simulink library "DAEMOT_Lib"  (R2019b)
settings: Solver=ode45  StartTime=0.0  StopTime=10.0  FixedStep=0.1  RelTol=1e-3
undefined symbols (not defined in the file or in its folder): Controller, CP, Ctrl, Ctrl_Fcn, Elec1, f, F2, Fluid, lag1, Mission, Moody, PropellerProp, rev_comms_sink
libraries: $bdroot x200, instrumentlib x21, simulink x5, dspsigops x2
(part 12 of 13)

== matlab function DAEMOT_Lib/Thermal/Heat Exchanger/HX ==
  data: x input; x_dot output; P_in input size=2; Mdot_down input size=2; Mdot input; T_in input size=2; H output; mu input size=2; k input size=2; Cp input size=2; Rho input size=2; E_fluid input size=2; M_wall parameter; Cp_wall parameter; Pass1 parameter; Pass2 parameter; f1 parameter; f2 parameter; KL1 parameter; KL2 parameter; b1 parameter; b2 parameter; W1 parameter; W2 parameter; L1 parameter; L2 parameter; Nu_lam1 parameter; Nu_lam2 parameter; dH1 parameter; dH2 parameter; HTC_method1 parameter; HTC_method2 parameter; HTC1 parameter; HTC2 parameter
function [x_dot,H]  = HX(x,P_in,Mdot_down,Mdot,T_in,mu,k,Cp,Rho,E_fluid,M_wall,Cp_wall,Pass1,Pass2,f1,f2,KL1,KL2,b1,b2,W1,W2,L1,L2,Nu_lam1,Nu_lam2,dH1,dH2,HTC_method1, HTC_method2, HTC1, HTC2)

% Parse data
P_in1       = P_in(1);
P_in2       = P_in(2);
Mdot_down1  = Mdot_down(1);
Mdot_down2  = Mdot_down(2);
Mdot1       = Mdot(1);
Mdot2       = Mdot(2);
T_in1       = T_in(1);
T_in2       = T_in(2);
mu1         = mu(1);
mu2         = mu(2);
k1          = k(1);
k2          = k(2);
Cp1         = Cp(1);
Cp2         = Cp(2);
Rho1        = Rho(1);
Rho2        = Rho(2);
E_fluid1    = E_fluid(1);
E_fluid2    = E_fluid(2);

% Constants and Conversions
Mdot_down1_pass = Mdot_down1/Pass1;
Mdot_down2_pass = Mdot_down2/Pass2;
Mdot1_pass = Mdot1/Pass1;
Mdot2_pass = Mdot2/Pass2;
g        = 9.81;                   % Gravitational acceleration [m/s^2]
A_ht1    = L1*(2*b1+2*W1);         % Heat transfer area
A_ht2    = L2*(2*b2+2*W2);         % Heat transfer area
V1       = L1*b1*W1;               % Volume per pass
V2       = L2*b2*W2;               % Volume per pass
Cp1      = 1000*Cp1;               % Convert Cp from J/g*K to J/kg*K
Cp2      = 1000*Cp2;               % Convert Cp from J/g*K to J/kg*K
k1       = 1000*k1;                % Convert k from kW/m*K to W/m*K
k2       = 1000*k2;                % Convert k from kW/m*K to W/m*K
C_wall   = M_wall*Cp_wall;         % Heat Capacitance (kJ/K)
C_wall   = 1000*C_wall;            % Covnert heat capacitance from kJ/K to J/K
D1       = 4*b1*W1/(2*b1+2*W1);    % Hydraulic diameter (side 1) (see Incropera, Eq. 8.66)
D2       = 4*b2*W2/(2*b2+2*W2);    % Hydraulic diameter (side 2) (see Incropera, Eq. 8.66)

% Parse states
Tw      = x(1);                 % Wall temperature
P1      = x(2);                 % Outlet pressure (side 1)
P2      = x(3);                 % Outlet pressure (side 2)
T1      = x(4);                 % Outlet temperature (side 1)
T2      = x(5);                 % Outlet temperature (side 2)

% Additional intermediate variable calculations
dP1         = (P_in1-P1)*1000;      % Pressure differential (side 1) [Pa]
dP2         = (P_in2-P2)*1000;      % Pressure differential (side 2) [Pa]
dP1         = dP1 + Rho1*g*dH1;     % Pressure differential corrected for hieght
dP2         = dP2 + Rho2*g*dH2;     % Pressure differential corrected for hieght
um1         = sign(dP1)*sqrt_Lip(2*abs(dP1)/(Rho1*(f1*L1/D1+KL1)));   % Fluid velocity (side 1) [m/s]
um2         = sign(dP2)*sqrt_Lip(2*abs(dP2)/(Rho2*(f2*L2/D2+KL2)));   % Fluid velocity (side 2) [m/s]
Re1         = Rho1*abs(um1)*D1/mu1;      % Reynolds number (side 1)
Re2         = Rho2*abs(um2)*D2/mu2;      % Reynolds number (side 1)
Pr1         = Cp1*mu1/k1;           % Prandtl number (side 1) (see Incropera, Table 6.2)
Pr2         = Cp2*mu2/k2;           % Prandtl number (side 2) (see Incropera, Table 6.2)

% Gneilinski
if Re1 < 2300
    Nu1 = Nu_lam1; % (inteprolated from Incropera, Table 8.1 in initialization)
else
    Nu1 = (f1/8)*(Re1-1000)*Pr1 / (1+12.7*(f1/8)^.5*(Pr1^(2/3)-1)); % (see Incropera, Eq. 8.62)
end
if Re2 < 2300
    Nu2 = Nu_lam2; % (inteprolated from Incropera, Table 8.1 in initialization)
else
    Nu2 = (f2/8)*(Re2-1000)*Pr2 / (1+12.7*(f2/8)^.5*(Pr2^(2/3)-1)); % (see Incropera, Eq. 8.62)
end

% Longo Correlation
% Nu1 = 0.277*Re1^0.766*Pr1^0.333;
% Nu2 = 0.277*Re2^0.766*Pr2^0.333;

% % Manglik Correlation
% Nu1 = 0.44*Re1^0.5*Pr1^0.333;
% Nu2 = 0.44*Re2^0.5*Pr2^0.333;

% Calculate outputs
if HTC_method1 == 0
    H1      = Nu1*k1/D1;        % Heat transfer coefficient (see Incropera, Table 6.2)
else
    H1 = HTC1;
end
if HTC_method2 == 0
    H2      = Nu2*k2/D2;        % Heat transfer coefficient (see Incropera, Table 6.2)
else
    H2 = HTC2;
end
H       = [H1 H2];

% Calculate state derivatives
Tw_dot = ( H1*A_ht1*(T1-Tw) + H2*A_ht2*(T2-Tw) )/C_wall;    % Wall temperature
P1_dot = (Mdot1_pass-Mdot_down1_pass)/(V1*Rho1/E_fluid1);   % Outlet pressure (side 1)
P2_dot = (Mdot2_pass-Mdot_down2_pass)/(V2*Rho2/E_fluid2);   % Outlet pressure (side 2)
Tout1_dot = (Mdot1_pass*(T_in1-T1)+H1*A_ht1/Cp1*(Tw-T1))/(V1*Rho1);   % Outlet temperature (side 1)
Tout2_dot = (Mdot2_pass*(T_in2-T2)+H2*A_ht2/Cp2*(Tw-T2))/(V2*Rho2);   % Outlet temperature (side 2)

% Mux state derivatives
x_dot  = [Tw_dot,P1_dot,P2_dot,Tout1_dot,Tout2_dot];

end

== matlab function DAEMOT_Lib/Legacy Components/Fluid Tank/Tank ==
  data: x input; x_dot output; Mdot_in input; Mdot_out input; T_in input; T_amb input; Cp input; M output; h output; Rho input; H parameter; D parameter; Pamb parameter
function [x_dot,M,h]= Tank(x,Mdot_in,Mdot_out,T_in,T_amb,Cp,Rho,H,D,Pamb)

% Constants and Conversions
A_cross = pi*D^2/4;             % Cross-sectional area
Cp      = 1000*Cp;              % Convert Cp from J/g*K to J/kg*K
g       = 9.81;                 % Gravitational acceleration

% Parse states
T      = x(1);                  % Temperature of the tank
P      = x(2);                  % Pressure at bottom of the tank

% Calculate outputs
h = 1000*(P-Pamb)/(Rho*g);      % Tank height
M = Rho*A_cross*h;              % Tank mass

% Additional intermediate variable calculations
A_ht    = pi*h*D;               % Heat transfer area          

% Calculate state derivatives
T_dot = (Mdot_in*(T_in-T)-H*A_ht*(T-T_amb)/Cp)/M;    % Tank temperature
P_dot  = (Mdot_in-Mdot_out)*g/(1000*A_cross);        % Tank pressure

% Mux state derivatives
x_dot  = [T_dot,P_dot];

end

== matlab function DAEMOT_Lib/Thermal/Pump/Pump ==
  data: x input; x_dot output; Mdot output; P_in input; T_in input; Power output; Mdot_down input; PWM input; E_fluid input; Rho input; D parameter; L parameter; t parameter; E parameter; v parameter; A input; H_k input; Rho_pump input; Eta_k input
function [x_dot,Mdot,Power]= Pump(x,P_in,T_in,Mdot_down,PWM,E_fluid,Rho,D,L,t,E,v,A,H_k,Rho_pump,Eta_k)


% Constants and Conversions
V           = L*pi*D^2/4;       % Volume
g           = 9.81;             % Gravitational acceleration

% Parse states
T       = x(1);                 % Temperature of the tank
P       = x(2);                 % Pressure at bottom of the tank

% Additional intermediate variable calculations
dP      = (P-P_in);             % Pressure difference [kPa]
PWM     = PWM/100;              % PWM in duty ratio [0-1]
H       = H_k' * [1; dP; PWM];   % Pump head [m]
Q       = sqrt_Lip( max(0,2*g*(H - 1000*dP/(Rho_pump*g))) )*A;  % Volumetric flow rate
WHP     = Rho*g*Q*H;            % Pump water horse power [W]
Eta     = Eta_k' * [1; WHP; PWM; WHP^2; PWM^2; WHP*PWM];   % Efficiency [%]

% Calculate outputs
Mdot    = Rho*Q;                % Mass flow rate [kg/s]
Power   = (Eta/100)*WHP;        % Pump electrical power [W]
         
% Calculate state derivatives
T_dot   = Mdot*(T_in-T)/(V*Rho);    % Pump outlet temperature 
P_dot   = (Mdot-Mdot_down)/(V*Rho*(1/E_fluid+D*(1-v/2)/(t*E))); % Pump outlet pressure

% Mux state derivatives
x_dot  = [T_dot,P_dot];

end

== matlab function DAEMOT_Lib/Legacy Components/Pipe_M_to_M/Pipe_M_to_M ==
  data: x input; x_dot output; Mdot_in input; Mdot_out input; Rho input; dRho_dP input; f input; D parameter; L parameter; P_in output; P_out output
function [x_dot,P_in,P_out] = Pipe_M_to_M(x,Mdot_in,Mdot_out,Rho,dRho_dP,f,D,L)

% Notes on Friction Factor:
% f is currently calculated using a lookup table generated with the "Hydro
% Scheme Designer" as: f  = moody(e/D,Re).  This Moody function
% automatically detects laminar vs. turbulent flow, but with a cutoff of 
% Re=2000.  This could lead to numerical issues in the future, as there is 
% a discrete transition in the lookup table at Re=2000 that could lead to
% oscillations about that point.

% Alternately, the code below could be used:
% f = (0.790*log(Re)-1.64)^-2; % (see Incropera, Eq. 8.21)
% if (Re<3000) || (Re>5*10^6)
%     disp('Reynolds Number is outside the range of the friction factor correlation.')
% end

mdot    = (Mdot_in+Mdot_out)/2; % Average mass flow rate
A_cross = pi*D^2/4;             % Cross-sectional area
V       = L*pi*D^2/4;           % Volume

% Parse states
P       = x(1);

% Calculate upstream and downstream pressure
L_diff  = L/2;
um      = mdot/(Rho*A_cross);
delta_P = (f*Rho*um^2/(2*D))*L_diff; % (see Incropera, Eq. 8.22a)
delta_P = delta_P/1000; % Convert from Pa to kPa
P_in    = P+delta_P;
P_out   = P-delta_P;

% Calculate state derivatives
P_dot   = (Mdot_in-Mdot_out)/(V*dRho_dP);

% Mux state derivatives
x_dot   = P_dot;

== matlab function DAEMOT_Lib/Thermal/Pipe_P_to_P/Pipe_P_to_M ==
  data: x_dot output; x input; T_in input; Mdot input; Rho input; D parameter; L parameter
function x_dot   = Pipe_P_to_M(x,T_in,Mdot,Rho,D,L)

% Constants and Conversions
V      = pi*D^2/4*L;            % Volume

% Parse states
T      = x(1);                  % Temperature of the tank

% Calculate state derivatives
T_dot  = Mdot*(T_in-T)/(V*Rho);  % Pipe outlet temperature

% Mux state derivatives
x_dot  = T_dot;

end

== matlab function DAEMOT_Lib/Thermal/Pipe_P_to_M/Pipe_P_to_M ==
  data: x_dot output; x input; T_in input; Mdot_down input; Mdot input; Rho input; E_fluid input; D parameter; L parameter; t parameter; E parameter; v parameter
function x_dot  = Pipe_P_to_M(x,T_in,Mdot_down,Mdot,Rho,E_fluid,D,L,t,E,v)

% Constants and Conversions
V       = L*pi*D^2/4;           % Volume

% Parse states
T       = x(1);                 % Temperature at the outlet of pipe
P       = x(2);                 % Pressure at the outlet of pipe

% Calculate state derivatives
T_dot = Mdot*(T_in-T)/(V*Rho);  % Pipe outlet temperature
P_dot = (Mdot-Mdot_down)/(V*Rho*(1/E_fluid+D*(1-v/2)/(t*E)));   % Pipe outlet pressure

% Mux state derivatives
x_dot  = [T_dot,P_dot];

end

== matlab function DAEMOT_Lib/Thermal/Pipe_P_to_M/Mdot ==
  data: P_in input; P_out input; Mdot output; Rho input; f parameter; D parameter; L parameter; KL parameter; dH parameter
function Mdot = Mdot(P_in,P_out,Rho,f,D,L,KL,dH)

% Constants and Conversions
g           = 9.81;                 % Gravitational acceleration [m/s^2]
A_cross     = pi*D^2/4;             % Cross sectional area
dP          = (P_in-P_out)*1000;    % Pressure differential [Pa]
dP          = dP + Rho*g*dH;        % Pressure differential corrected for hieght
um          = max(0,sign(dP)*sqrt_Lip(2*abs(dP)/(Rho*(f*L/D+KL))));    % Fluid velocity [m/s]

% Calculate outputs
Mdot        = um*Rho*A_cross;       % Mass flow rate [kg/s]

end

== matlab function DAEMOT_Lib/Legacy Components/Pipe_M_to_P/Pipe_P_to_M ==
  data: x_dot output; x input; P_out input; Mdot_up input; Mdot output; Rho input; dRho_dP input; f input; D parameter; L parameter
function [x_dot,Mdot]  = Pipe_P_to_M(x,P_out,Mdot_up,Rho,dRho_dP,f,D,L)

% Notes on Friction Factor:
% f is currently calculated using a lookup table generated with the "Hydro
% Scheme Designer" as: f  = moody(e/D,Re).  This Moody function
% automatically detects laminar vs. turbulent flow, but with a cutoff of 
% Re=2000.  This could lead to numerical issues in the future, as there is 
% a discrete transition in the lookup table at Re=2000 that could lead to
% oscillations about that point.

% Alternately, the code below could be used:
% f = (0.790*log(Re)-1.64)^-2; % (see Incropera, Eq. 8.21)
% if (Re<3000) || (Re>5*10^6)
%     disp('Reynolds Number is outside the range of the friction factor correlation.')
% end

% Perform various conversions
A_cross = pi*D^2/4;                % Cross-sectional area
V       = L*pi*D^2/4;              % Volume

% Parse states
P_in  = x;

% Calculate mass flow rate
dP       = (P_in-P_out)*1000;
um       = sign(dP)*sqrt(4*abs(dP)*D/(L*Rho*f));
Mdot     = um*Rho*A_cross;

% Calculate state derivatives
P_dot  = (Mdot_up-Mdot)/(V*dRho_dP);

% Mux state derivatives
x_dot  = P_dot;

== matlab function DAEMOT_Lib/Thermal/Pipe_P_to_P/Mdot ==
  data: P_in input; P_out input; Mdot output; Rho input; f parameter; D parameter; L parameter; KL parameter; dH parameter
function Mdot = Mdot(P_in,P_out,Rho,f,D,L,KL,dH)

% Constants and Conversions
g           = 9.81;                 % Gravitational acceleration [m/s^2]
A_cross     = pi*D^2/4;             % Cross sectional area
dP          = (P_in-P_out)*1000;    % Pressure differential [Pa]
dP          = dP + Rho*g*dH;        % Pressure differential corrected for hieght
um          = max(0,sign(dP)*sqrt_Lip(2*abs(dP)/(Rho*(f*L/D+KL))));    % Fluid velocity [m/s]

% Calculate outputs
Mdot        = um*Rho*A_cross;       % Mass flow rate [kg/s]

end

== matlab function DAEMOT_Lib/Thermal/Heat Exchanger/Mdot ==
  data: P_in1 input; P_in2 input; Mdot1_tot output; P_out1 input; P_out2 input; Rho1 input; Rho2 input; f1 parameter; f2 parameter; b1 parameter; b2 parameter; W1 parameter; W2 parameter; L1 parameter; L2 parameter; KL1 parameter; KL2 parameter; Mdot2_tot output; Pass1 parameter; Pass2 parameter; dH1 parameter; dH2 parameter
function [Mdot1_tot,Mdot2_tot]   = Mdot(P_in1,P_in2,P_out1,P_out2,Rho1,Rho2,f1,f2,b1,b2,W1,W2,L1,L2,KL1,KL2,Pass1,Pass2,dH1,dH2)

% Constants and Conversions
g           = 9.81;                 % Gravitational acceleration [m/s^2]
D1 = 4*b1*W1/(2*b1+2*W1);           % (see Incropera, Eq. 8.66)
D2 = 4*b2*W2/(2*b2+2*W2);           % (see Incropera, Eq. 8.66)
dP1         = (P_in1-P_out1)*1000;  % Pressure differential (side 1) [Pa]
dP2         = (P_in2-P_out2)*1000;  % Pressure differential (side 2) [Pa]
dP1         = dP1 + Rho1*g*dH1;     % Pressure differential corrected for hieght
dP2         = dP2 + Rho2*g*dH2;     % Pressure differential corrected for hieght
um1         = max(0,sign(dP1)*sqrt_Lip(2*abs(dP1)/(Rho1*(f1*L1/D1+KL1)))); % Fluid velocity (side 1) [m/s]
um2         = max(0,sign(dP2)*sqrt_Lip(2*abs(dP2)/(Rho2*(f2*L2/D2+KL2)))); % Fluid velocity (side 2) [m/s]
Mdot1_pass  = um1*Rho1*b1*W1;       % Mass flow rate per pass (side 1) [kg/s]
Mdot2_pass  = um2*Rho2*b2*W2;       % Mass flow rate per pass (side 2) [kg/s]

% Calculate outputs
Mdot1_tot = Mdot1_pass*Pass1;       % Total mass flow rate (side 1) [kg/s]
Mdot2_tot = Mdot2_pass*Pass2;       % Total mass flow rate (side 2) [kg/s]

end

== matlab function DAEMOT_Lib/Legacy Components/Pipe_P_to_M1/Mdot ==
  data: P_in input; P_out input; Mdot output; Rho input; f parameter; D parameter; L parameter; KL parameter; dH parameter
function Mdot = Mdot(P_in,P_out,Rho,f,D,L,KL,dH)

% Constants and Conversions
g           = 9.81;                 % Gravitational acceleration [m/s^2]
A_cross     = pi*D^2/4;             % Cross sectional area
dP          = (P_in-P_out)*1000;    % Pressure differential [Pa]
dP          = dP + Rho*g*dH;        % Pressure differential corrected for hieght
um          = sign(dP)*sqrt(2*abs(dP)/(Rho*(f*L/D+KL)));    % Fluid velocity [m/s]

% Calculate outputs
Mdot        = um*Rho*A_cross;       % Mass flow rate [kg/s]

end

== matlab function DAEMOT_Lib/Legacy Components/Pipe_P_to_M1/Pipe_P_to_M ==
  data: x_dot output; x input; T_in input; Mdot_down input; Mdot input; Rho input; E_fluid input; D parameter; L parameter; t parameter; E parameter; v parameter
function x_dot  = Pipe_P_to_M(x,T_in,Mdot_down,Mdot,Rho,E_fluid,D,L,t,E,v)

% Constants and Conversions
V      = pi*D^2/4*L;            % Volume

% Parse states
T       = x(1);                 % Temperature at the outlet of pipe
P       = x(2);                 % Pressure at the outlet of pipe

% Calculate state derivatives
T_dot = Mdot*(T_in-T)/(V*Rho);  % Pipe outlet temperature
P_dot = (Mdot-Mdot_down)/(V*Rho*(1/E_fluid+D*(1-v/2)/(t*E)));   % Pipe outlet pressure

% Mux state derivatives
x_dot  = [T_dot,P_dot];

end

== matlab function DAEMOT_Lib/Legacy Components/Pipe_P_to_P1/Mdot ==
  data: P_in input; P_out input; Mdot output; Rho input; f parameter; D parameter; L parameter; KL parameter; dH parameter
function Mdot = Mdot(P_in,P_out,Rho,f,D,L,KL,dH)

% Constants and Conversions
g           = 9.81;                 % Gravitational acceleration [m/s^2]
A_cross     = pi*D^2/4;             % Cross sectional area
dP          = (P_in-P_out)*1000;    % Pressure differential [Pa]
dP          = dP + Rho*g*dH;        % Pressure differential corrected for hieght
um          = sign(dP)*sqrt(2*abs(dP)/(Rho*(f*L/D+KL)));    % Fluid velocity [m/s]

% Calculate outputs
Mdot        = um*Rho*A_cross;       % Mass flow rate [kg/s]

end

== matlab function DAEMOT_Lib/Legacy Components/Pipe_P_to_P1/Pipe_P_to_M ==
  data: x_dot output; x input; T_in input; Mdot input; Rho input; D parameter; L parameter
function x_dot   = Pipe_P_to_M(x,T_in,Mdot,Rho,D,L)

% Constants and Conversions
V      = pi*D^2/4*L;            % Volume

% Parse states
T      = x(1);                  % Temperature of the tank

% Calculate state derivatives
T_dot  = Mdot*(T_in-T)/(V*Rho);  % Pipe outlet temperature

% Mux state derivatives
x_dot  = T_dot;

end

== matlab function DAEMOT_Lib/Legacy Components/Solenoid_P_to_P/Mdot ==
  data: P_in input; P_out input; Mdot output; Rho input; f parameter; D parameter; L parameter; KL parameter
function Mdot = Mdot(P_in, P_out, Rho, f, D, L, KL)

% Constants and Conversions
A_cross     = pi*D^2/4;             % Cross sectional area
dP          = (P_in-P_out)*1000;    % Pressure differential [Pa]
um          = max(1e-6,sign(dP)*sqrt_Lip(2*abs(dP)/(Rho*(f*L/D+KL))));    % Fluid velocity [m/s]

% Calculate outputs
Mdot        = um*Rho*A_cross;       % Mass flow rate [kg/s]

end

== matlab function DAEMOT_Lib/Legacy Components/Solenoid_P_to_P/Pipe_P_to_M ==
  data: x_dot output; x input; T_in input; Mdot input; Rho input; D parameter; L parameter
function x_dot   = Solenoid_P_to_P(x,T_in,Mdot,Rho,D,L)

% Constants and Conversions
V      = pi*D^2/4*L;            % Volume

% Parse states
T      = x(1);                  % Temperature of the tank

% Calculate state derivatives
T_dot  = Mdot*(T_in-T)/(V*Rho);  % Pipe outlet temperature

% Mux state derivatives
x_dot  = T_dot;

end

== matlab function DAEMOT_Lib/Legacy Components/Solenoid_P_to_M/Mdot ==
  data: P_in input; P_out input; Mdot output; Rho input; f parameter; D parameter; L parameter; KL parameter
function Mdot = Mdot(P_in,P_out,Rho,f,D,L,KL)

% Constants and Conversions
A_cross     = pi*D^2/4;             % Cross sectional area
dP          = (P_in-P_out)*1000;    % Pressure differential [Pa]
um          = max(1e-6,sign(dP)*sqrt_Lip(2*abs(dP)/(Rho*(f*L/D+KL))));    % Fluid velocity [m/s]

% Calculate outputs
Mdot        = um*Rho*A_cross;       % Mass flow rate [kg/s]

end

== matlab function DAEMOT_Lib/Legacy Components/Solenoid_P_to_M/Pipe_P_to_M ==
  data: x_dot output; x input; T_in input; Mdot_down input; Mdot input; Rho input; E_fluid input; D parameter; L parameter; t parameter; E parameter; v parameter
function x_dot  = Solenoid_P_to_M(x,T_in,Mdot_down,Mdot,Rho,E_fluid,D,L,t,E,v)

% Constants and Conversions
V       = L*pi*D^2/4;           % Volume

% Parse states
T       = x(1);                 % Temperature at the outlet of pipe
P       = x(2);                 % Pressure at the outlet of pipe

% Calculate state derivatives
T_dot = Mdot*(T_in-T)/(V*Rho);  % Pipe outlet temperature
P_dot = (Mdot-Mdot_down)/(V*Rho*(1/E_fluid+D*(1-v/2)/(t*E)));   % Pipe outlet pressure

% Mux state derivatives
x_dot  = [T_dot,P_dot];

end

== matlab function DAEMOT_Lib/Thermal/Multi-Port Fluid Tank/Tank ==
  data: x input; x_dot output; Mdot_in input; Mdot_out input; T_in input; T_amb input; Cp input; M output; h output; Rho input; H parameter; D parameter; Pamb parameter
function [x_dot,M,h]= Tank(x,Mdot_in,Mdot_out,T_in,T_amb,Cp,Rho,H,D,Pamb)

% Constants and Conversions
Mdot_in_tot     = sum(Mdot_in);     % Total mass flow rate in
Mdot_out_tot    = sum(Mdot_out);    % Total mass flow rate out
A_cross = pi*D^2/4;             % Cross-sectional area
Cp      = 1000*Cp;              % Convert Cp from J/g*K to J/kg*K
g       = 9.81;                 % Gravitational acceleration

% Parse states
T      = x(1);                  % Temperature of the tank
P      = x(2);                  % Pressure at bottom of the tank

% Calculate outputs
h = 1000*(P-Pamb)/(Rho*g);      % Tank height
M = Rho*A_cross*h;              % Tank mass

% Additional intermediate variable calculations
A_ht    = pi*h*D;               % Heat transfer area          

% Calculate state derivatives
T_dot = ((dot(Mdot_in,T_in)-sum(Mdot_in)*T)-H*A_ht*(T-T_amb)/Cp)/M;    % Tank temperature
P_dot  = (Mdot_in_tot-Mdot_out_tot)*g/(1000*A_cross);        % Tank pressure

% Mux state derivatives
x_dot  = [T_dot,P_dot];

end

== matlab function DAEMOT_Lib/Legacy Components/Generator/Generator ==
  data: Omega input; I input; Torque output; V parameter; eta parameter; Q output
function [Torque,Q]   = Generator(Omega,I,V,eta)

% Constants and Conversions

% Parse states

% Additional intermediate variable calculations

% Calculate outputs
Torque = 1/(Omega*eta)*I*V;     % Generator torque (Nm)
Q = (1-eta)*Torque*Omega/1000;       % Generator heat (kW)

% Calculate state derivatives

% Mux state derivatives

end

== matlab function DAEMOT_Lib/Legacy Components/Aircraft/Aircraft ==
  data: x input; x_dot output; Thrust_1 input; Thrust_2 input; M_fuel input; M_dry parameter; M_load parameter; rho parameter; A parameter; Cd parameter
function x_dot = Aircraft(x,Thrust_1,Thrust_2,M_fuel,M_dry, M_load, rho, A, Cd)

% Parse states
Vel      = x(1);                  % Velocity of aircraft

% Additional intermediate variable calculations
M_tot  = M_fuel+M_dry+M_load;   % Total mass
Drag   = 0.5*rho*A*Cd*Vel^2;      % Drag force

% Calculate state derivatives
V_dot  = 1/(M_tot)*(Thrust_1+Thrust_2-Drag);    % Velocity

% Mux state derivatives
x_dot  = [V_dot];

end

== matlab function DAEMOT_Lib/Legacy Components/Engine/Engine ==
  data: x input; Mdot input; Vel input; Torque input; U input; x_dot output; Thrust output; J parameter; Thrust_max parameter; Omega_max parameter; Q_bearings output; alpha parameter; eta parameter
function [x_dot,Thrust,Q_bearings]  = Engine(x,Mdot,Vel,Torque,U,J,Thrust_max,Omega_max, alpha, eta)

% Constants and Conversions

% Parse states
Omega     = x(1);                 % Shaft Speed

% Additional intermediate variable calculations

% Calculate outputs
Thrust    = Thrust_max*(Omega/Omega_max)^3;  % Engine Thrust [N]
Q_burn    = (1-eta)*U*Mdot;           % Heat generation (leaves engine with exhaust) [kW]
Q_bearings = alpha*Omega;               % Bearing heat generation (cooled by oil) [kW]

% Calculate state derivatives
Omega_dot = 1/(J*Omega)*(1000*U*Mdot-Thrust*Vel-Torque*Omega-1000*(Q_burn+Q_bearings));    % Shaft speed 

% Mux state derivatives
x_dot  = [Omega_dot];

end

== matlab function DAEMOT_Lib/Thermal/Peristaltic_Pump/MATLAB Function ==
  data: P input; mdot output; w input; H_k input
% Calibration equations for drain pump 1 and drain pump 2 operating
% together at the same pump speed
% See 'Peristaltic Pump Flow Rates New Config.xlsx'

% mdot, kg/s - combined mass flow rate through both drain pumps
% w, [0-10] - drain pump speed (both drain pumps operate at same speed
% P, kPa - pressure at drain pumps

% Map for mdot was created Support Functions folder and raw data is
% in sensor calibration folder

function mdot = DrainPump(P, w, H_k)

mdot = any(w)*H_k(1) + H_k(2)*w + any(w)*H_k(3)*P;

% mdot = -0.0003743277602398326 + 0.00015072862953603*w + ...
%     0.00000307012873321525*P;
    
end

== matlab function DAEMOT_Lib/Legacy Components/Battery/Battery ==
  data: x input; V_in input; P input; x_dot output; I_in output; Q output; eta input; C parameter
function [x_dot,I_in,Q]  = Battery(x,V_in,P,eta,C)

% Constants and Conversions

% Parse states
SOC     = x(1);                 % State of charge

% Additional intermediate variable calculations

% Calculate outputs
if P >= 0   % Charge mode
    P_in = 1/eta*P;
    Q = (1-eta)*P_in;
else        % Discharge mode
    P_in = eta*P;
    Q = -(1-eta)*P;
end
I_in = 1000*P_in/V_in;

% Calculate state derivatives
SOC_dot = 1/(1000*C)*P;    % State of charge

% Mux state derivatives
x_dot  = [SOC_dot];

end

== matlab function DAEMOT_Lib/Electrical/Battery/Electrical ==
  data: I input; V input; T_m input; V1_dot output; props input size=[1 7]; B_cap parameter; V2_dot output; SOC_dot output; V_T output; Q output; Np parameter; Ns parameter
function [V1_dot,V2_dot,SOC_dot,V_T,Q]= Electrical(I,V,T_m,props,B_cap, Np,Ns)
%% Electrical Effects Function
Rs = props(1)*Ns/Np;
R1 = props(2)*Ns/Np;
C1 = props(3)*Np/Ns;
R2 = props(4)*Ns/Np;
C2 = props(5)*Np/Ns;
dU_dt = props(6)*Ns;
V_ocv = props(7);
V1 = V(1);
V2 = V(2);
%outputs = zeros(1,5);

%% Voltage Dynamics
V1_dot = -V1/(R1*C1) + I/C1;
V2_dot = -V2/(R2*C2) + I/C2;

%% State of Charge Dynamic
SOC_dot = -I/(3600*B_cap*Np);

%% Terminal Voltage
V_T = V_ocv - V1 - V2 - I*Rs;

%% Heat Generation
Q_s = (T_m+273)*dU_dt/1000; %entropic heat
Q = I^2*Rs + V1^2/R1 + V2^2/R2 - I*Q_s/Np;

== matlab function DAEMOT_Lib/Legacy Components/Converter/Converter ==
  data: V_in input; I input; I_in output; V parameter; I0 parameter; Q output; eta_max parameter; eta_min parameter; eta output
function [I_in,Q,eta]   = Converter(V_in,I,V,I0,eta_max, eta_min)

% Constants and Conversions

% Parse states

% Additional intermediate variable calculations
a = -(eta_max-eta_min)/I0^2;
b = 2*(eta_max-eta_min)/I0;
c = eta_min;
eta = a*I^2 + b*I + c;

% Calculate outputs
if V_in > 0
    I_in = 1/(V_in*eta)*I*V;     % Converter torque (Nm)
else
    I_in = 0;
end
Q = (1-eta)*I_in*V_in/1000;       % Converter heat (kW)

% Calculate state derivatives

% Mux state derivatives

end

== matlab function DAEMOT_Lib/Legacy Components/Pump/Pump ==
  data: x input; x_dot output; Mdot output; P_in input; T_in input; V_in input; I output; Mdot_down input; Omega input; E parameter; D parameter; L parameter; Omega_max parameter; DP_max parameter; mdot_max parameter; Q output; alpha parameter; eta output; rho input; cp input
function [x_dot,Mdot,I,Q,eta]= Pump(x,P_in,T_in,V_in,Mdot_down,Omega,E,D,L,Omega_max,DP_max,mdot_max,alpha, rho, cp)

coder.extrinsic('gcb')
% Constants and Conversions
Vol           = L*pi*D^2/4;       % Volume

% Parse states
T       = x(1);                 % Outlet fluid temperature
P       = x(2);                 % Outlet fluid pressure

% Additional intermediate variable calculations
dP      = (P-P_in);             % Pressure difference [kPa]
lambda  = Omega/Omega_max;      % Fraction of max shaft speed [-]
a       = -DP_max/(lambda*mdot_max^2);      % Pump map parameters
c       = lambda*DP_max;                    % Pump map parameters


% Calculate outputs
Q       = alpha*Omega;                       % Heat generation [kW]
if Omega > 0
    Mdot    = max(0,sqrt_Lip((dP-c)/a));                % Mass flow rate [kg/s]
    I       = 1000/V_in*(Mdot*dP/rho+Q);       % Inlet current [A]
    eta     = 1000*(Mdot*dP/rho)/(I*V_in);
else
    Mdot    = 0;                % Mass flow rate [kg/s]
    I       = 0;
    eta     = 0;
end
     
if Omega > Omega_max || (P - P_in) > DP_max || Mdot > mdot_max
%      warning(['Violated maximum values for pump. See ',gcb])
end
% Calculate state derivatives
T_dot   = Mdot*(T_in-T)/(Vol*rho)+Q/(Vol*rho*cp);   % Pump outlet temperature 
P_dot   = (Mdot-Mdot_down)/(Vol*rho/E);     % Pump outlet pressure

% Mux state derivatives
x_dot  = [T_dot,P_dot];

end

== matlab function DAEMOT_Lib/Legacy Components/Fan/Pump ==
  data: x input; x_dot output; Mdot output; P_in input; T_in input; V_in input; I output; Mdot_down input; Omega input; E parameter; D parameter; L parameter; Omega_max parameter; DP_max parameter; mdot_max parameter; Q output; alpha parameter; eta output; cp input; rho input
function [x_dot,Mdot,I,Q,eta]= Pump(x,P_in,T_in,V_in,Mdot_down,Omega,E,D,L,Omega_max,DP_max,mdot_max,alpha, cp, rho)


% Constants and Conversions
Vol           = L*pi*D^2/4;       % Volume

% Parse states
T       = x(1);                 % Outlet fluid temperature
P       = x(2);                 % Outlet fluid pressure

% Additional intermediate variable calculations
dP      = (P-P_in);             % Pressure difference [kPa]
lambda  = Omega/Omega_max;      % Fraction of max shaft speed [-]
a       = -DP_max/(lambda*mdot_max^2);      % Pump map parameters
c       = lambda*DP_max;                    % Pump map parameters

% Calculate outputs
Q       = alpha*Omega;                       % Heat generation [kW]
if Omega > 0
    Mdot    = max(0,sqrt_Lip((dP-c)/a));                % Mass flow rate [kg/s]
    I       = 1000/V_in*(Mdot*dP/rho+Q);       % Inlet current [A]
    eta     = 1000*(Mdot*dP/rho)/(I*V_in);
else
    Mdot    = 0;                % Mass flow rate [kg/s]
    I       = 0;
    eta     = 0;
end
         
% Calculate state derivatives
T_dot   = Mdot*(T_in-T)/(Vol*rho)+Q/(Vol*rho*cp);   % Pump outlet temperature 
P_dot   = (Mdot-Mdot_down)/(Vol*rho/E);     % Pump outlet pressure

% Mux state derivatives
x_dot  = [T_dot,P_dot];

end

== matlab function DAEMOT_Lib/Electrical/Battery/Thermal ==
  data: Q input; Tc_dot output; T input; Q_sink input; C_c parameter; C_s parameter; R_cond parameter; Ts_dot output; Ns parameter; Np parameter
function [Tc_dot,Ts_dot]= Thermal(Q,T,Q_sink,C_c, C_s, R_cond, Ns, Np)
%% Thermal Effects Function
T_c = T(1);
T_s = T(2);

%% Core Temperature Dynamic
Tc_dot = (Q + Ns*Np*(T_s-T_c)/R_cond)/(Np*Ns*C_c);

%% Surface Temperature Dynamic
Ts_dot = (Ns*Np*(T_c-T_s)/R_cond - Q_sink)/(Np*Ns*C_s);

== matlab function DAEMOT_Lib/Electrical/Resistor/Electrical ==
  data: V_in input; out output; in input; R input; r_type parameter; Q output
function [out,Q]= voltage(V_in, in, R, r_type)
%% Output 

if r_type == 1 %voltage type
    out = (V_in - in)/R;
    Q = (V_in - in)/R^2;
else %current type
    out = V_in - in*R;
    Q = R^2*in;
end

== matlab function DAEMOT_Lib/Electrical/Resistor/Thermal ==
  data: Q input; T_dot output; Q_sink input; Cp parameter
function T_dot = Thermal(Q, Q_sink, Cp)
%% Load Temperature
T_dot = (1/Cp) * (Q - Q_sink);

== matlab function DAEMOT_Lib/Thermal/Air Volume/Air_Volume ==
  data: x input; x_dot output; Mdot_in input; Mdot_out input; T_in input; T_amb input; Cp input; Rho input; Q input; H parameter; D parameter; A_sa parameter; V parameter; E_fluid parameter
function x_dot = Air_Volume(x,Mdot_in,Mdot_out,T_in,T_amb,Cp,Rho,Q,H,D,A_sa,V,E_fluid)

% Constants and Conversions
A_cross = pi*D^2/4;             % Cross-sectional area
Cp      = 1000*Cp;              % Convert Cp from J/g*K to J/kg*K
g       = 9.81;                 % Gravitational acceleration

% Parse states
T      = x(1);                  % Temperature of the tank
P      = x(2);                  % Pressure at bottom of the tank
M      = x(3);                  % Pressure at bottom of the tank

% Calculate outputs
% h = 1000*(P-Pamb)/(Rho*g);      % Tank height
% M = Rho*A_cross*h;              % Tank mass

% Additional intermediate variable calculations
% A_ht    = pi*h*D;               % Heat transfer area          
A_ht = A_sa;

% Calculate state derivatives
T_dot = (Mdot_in*(T_in-T)-H*A_ht*(T-T_amb)/Cp + Q/Cp)/M; % Tank temperature
P_dot  = (Mdot_in-Mdot_out)/(V*Rho*(1/E_fluid));        % Tank pressure
% M_dot = (Mdot_in-Mdot_out);

% Mux state derivatives
x_dot  = [T_dot,P_dot,0];

end

== matlab function DAEMOT_Lib/Electrical/Motor/Current ==
  data: V_in input; I_in input; Kv parameter; R parameter; L parameter; omega input; dI_dt output; Q_elec output
function [dI_dt,Q_elec]= current(V_in,I_in,Kv, R, L,omega)


dI_dt = (1/L) * (V_in - R*I_in - Kv*omega);

Q_elec = R*I_in^2;

== matlab function DAEMOT_Lib/Electrical/Motor/Omega ==
  data: I_in input; T_load input; omega_dot output; Kv parameter; omega input; T_motor output; J parameter; b parameter; c parameter; Q_mech output
function [omega_dot,T_motor,Q_mech]= omega(I_in,T_load,Kv,omega,J, b,c)

T_motor = Kv*I_in;

omega_dot = (1/(J))*(T_motor - T_load - b*omega - c*(2./(1+exp(-5*omega)) - 1));
Q_mech = b*omega^2 + c*omega*(2./(1+exp(-5*omega)) - 1);

== matlab function DAEMOT_Lib/Electrical/Motor/Thermal ==
  data: Q_elec input; Q_mech input; T_dot output; Q_sink input; Cp parameter
function T_dot = Thermal(Q_elec,Q_mech, Q_sink, Cp)
%% Load Temperature
T_dot = (1/Cp) * (Q_elec + Q_mech - Q_sink);

== matlab function DAEMOT_Lib/Electrical/Converter/Current ==
  data: I_out input; D input; I_in output; s input; dir parameter
function I_in = current(I_out,D,s,dir)

if dir == 1 %Boost ===>
    if s == 0     % Buck Mode
        I_in = I_out/D;
    else    % Boost Mode
        I_in = I_out/(1-D);
    end
elseif dir == 2 %Boost <===
    if s == 0     % Buck Mode
        I_in = D*I_out;
    else    % Boost Mode
        I_in = (1-D)*I_out;
    end
end

== matlab function DAEMOT_Lib/Electrical/Capacitor/Voltage ==
  data: I_in input; V_dot output; I_out input; C parameter
function V_dot = voltage(I_in, I_out,C)

V_dot = (1/C) * (I_in-I_out);

== matlab function DAEMOT_Lib/Electrical/Converter/Thermal ==
  data: Q input; T_dot output; Q_sink input; Cp parameter
function T_dot = Thermal(Q, Q_sink, Cp)
%% Load Temperature
T_dot = (1/Cp) * (Q - Q_sink);

== matlab function DAEMOT_Lib/Electrical/Converter/Voltage ==
  data: V_in input; V_out output; I_in input; I_out input; D input; s input; V_D parameter; R_D parameter; R_s parameter; R_L parameter; Q output; dir parameter
function [V_out,Q]= voltage(V_in,I_in,I_out,D,s,V_D, R_D, R_s, R_L,dir)

if dir == 1 %Boost ===>
    I_L = I_in;
    if s == 0     % Buck Mode
        V_out = (1/D) * (V_in - R_L*I_L - D*R_s*I_L - (1-D)*R_D*I_L + (1-D)*V_D);
        Q = (1/D)^2 * (R_L*I_out^2 + D*R_s*I_out^2 + (1-D)*R_D*I_out^2);
    else    % Boost Mode
        V_out = (1/(1-D)) * (V_in - R_L*I_L - D*R_s*I_L - (1-D)*R_D*I_L - (1-D)*V_D);
        Q = (1/(1-D))^2 * (R_L*I_out^2 + D*R_s*I_out^2 + (1-D)*R_D*I_out^2);
    end
elseif dir == 2 %Boost <===
    I_L = I_out;
    if s == 0     % Buck Mode
        V_out = D*V_in - D*R_s*I_L - R_L*I_L - (1-D)*V_D - (1-D)*R_D*I_L;
        Q = (R_L*I_out^2 + D*R_s*I_out^2 + (1-D)*R_D*I_out^2);
    else    % Boost Mode
        V_out = (1-D)*V_in - D*R_s*I_L - R_L*I_L + (1-D)*V_D - (1-D)*R_D*I_L;
        Q = (R_L*I_out^2 + D*R_s*I_out^2 + (1-D)*R_D*I_out^2);
    end
end

== matlab function DAEMOT_Lib/Electrical/Bus/current ==
  data: Iin_dot output; V_in input; V_out input; I_in input; I_out input; u_in input; u_out input; L parameter; R parameter; Iout_bar output
function [Iin_dot,Iout_bar]= current(V_in,V_out,I_in,I_out,u_in,u_out, L,R)
%% Input Current

Iin_dot = (1/L) * ((V_in - V_out).*u_in - I_in*R);
Iout_bar = u_out'*I_out;

== matlab function DAEMOT_Lib/Electrical/Bus/voltage ==
  data: I_in input; Ibar_out input; V_dot output; C parameter
function V_dot = voltage(I_in,Ibar_out,C)
%% Output Voltage

Ibar_in = sum(I_in);
V_dot = (Ibar_in - Ibar_out)/C;

== matlab function DAEMOT_Lib/Electrical/Voltage Bus/current ==
  data: I_out input; u input; I_in output
function I_in = Current(I_out,u)
%% Input Current
I_in = u'*I_out;

%I_in = (V_in-V_out)/R_i;

== matlab function DAEMOT_Lib/Electrical/Voltage Bus/voltage ==
  data: V_in input; V_out output; u input
function V_out = Voltage(V_in,u)
%% Output Voltage

V_out = V_in.*u;

% if Gn == 1
%     V_dot = 0;
% else
%     V_dot = (I_in-sum(I_out))/G_cap;
% end

== matlab function DAEMOT_Lib/Electrical/Inverter_v1/Thermal ==
  data: Q input; T_dot output; Q_sink input; Cp parameter
function T_dot = Thermal(Q, Q_sink, Cp)
%% Load Temperature
T_dot = (1/Cp) * (Q - Q_sink);

== matlab function DAEMOT_Lib/Electrical/Inductor/Current ==
  data: V_in input; V_out input; dI_dt output; L parameter
function dI_dt = current(V_in, V_out,L)

dI_dt = (V_in-V_out)/L;

== matlab function DAEMOT_Lib/Electrical/Inverter_v1/Voltage_Current ==
  data: V_in input; I_out input; D input; V_out output; I_in output; R3 parameter; Q output; R1 parameter; R2 parameter
function [V_out,I_in,Q]= voltage_current(V_in,I_out,D,R3, R1, R2)

I_in = (D^2*V_in + R3*I_out) / (D*R2 + R3);
V_out = (D*R3*V_in - R2*R3*I_out) / (D*R2 + R3);

Q = D*V_in^2/R1 + R2*I_in^2 + D*V_out^2/R2;

== matlab function DAEMOT_Lib/Electrical/Generator/Voltage1 ==
  data: V_in input; I output; u input; G parameter; cI parameter; cSFC parameter; mu_V parameter; std_V parameter; mu_u parameter; std_u parameter; S output
function [I,S]= voltage(V_in, u, G, cI, cSFC, mu_V, std_V, mu_u, std_u)
%% Output V_normoltage

u_norm = (u - mu_u)/std_u; %normalize
V_norm = (V_in - mu_V)/std_V; %normalize

I = -G * (cI(1) + cI(2)*V_norm + cI(3)*u_norm + ...
     cI(4)*V_norm*u_norm + cI(5)*u_norm.^2 + cI(6)*V_norm*u_norm.^2 +...
     cI(7)*u_norm.^3 + cI(8)*V_norm*u_norm.^3 + cI(9)*u_norm.^4);

S = (cSFC(1) + cSFC(2)*V_norm + cSFC(3)*u_norm + ...
     cSFC(4)*V_norm*u_norm + cSFC(5)*u_norm.^2 + cSFC(6)*V_norm*u_norm.^2 +...
     cSFC(7)*u_norm.^3 + cSFC(8)*V_norm*u_norm.^3 + cSFC(9)*u_norm.^4);
 
if V_in < 40
    I = 0;
    S = 0;
end

== matlab function DAEMOT_Lib/Electrical/UAV/speed ==
  data: v input; omega input; props input size=4; rho parameter; d parameter; b parameter; dv_dt output; tau output; m parameter
function [dv_dt,tau]= speed(v,omega,props,rho,d,b,m)

C_T = props(2);
C_L = props(3);
eta_prop = props(4); 
% C_T = .06;

dv_dt = (1/m) * (rho*(omega/(2*pi))^2*d^4*C_T - b*v);
% tau = rho*(omega/(2*pi))^2*d^5*C_L*eta_prop;
tau = v*omega*rho*(1/(2*pi))^2*d^4*C_T;

== matlab function DAEMOT_Lib/Electrical/Ground Vehicle/Torque ==
  data: omega input; t_load output; R parameter; rho_air parameter; Cd parameter; Af parameter; t_brake input; v output
function [t_load,v]= torque(omega, R, rho_air, Cd, Af,t_brake)

t_drive = .5*rho_air*Cd*Af*(omega*R)^2;

t_load = t_drive + t_brake;
v = omega*R;

== matlab function DAEMOT_Lib/Thermal/Heat_Sink_Edge/Thermal ==
  data: T_source input; T_sink input; k parameter; As parameter; Q output; s parameter; L parameter; R_const parameter
function Q = Thermal(T_source, T_sink, k, As, s, L, R_const )
%% Thermal Effects Function
%Assume 1-D conduction through a plane wall

if s == 0
    R = L/(k*As);
else
    R = R_const;
end
Q = (1/R) * (T_source - T_sink)/1000;

== matlab function DAEMOT_Lib/Thermal/Cold_Plate/Cold_Plate ==
  data: x input; Q_load input; x_dot output; P_in input; Mdot_down input; Mdot input; T_in input; H output; mu input; k input; Cp input; Rho input; E_fluid input; f parameter; M_wall parameter; Cp_wall parameter; D parameter; L parameter; t parameter; E parameter; v parameter; KL parameter; dH parameter; PAF parameter; Re output; HTC_method parameter; HTC parameter
function [x_dot,H,Re]  = Cold_Plate(x,Q_load,P_in,Mdot_down,Mdot,T_in,mu,k,Cp,Rho,E_fluid,f,M_wall,Cp_wall,D,L,t,E,v,KL,dH,PAF,HTC_method, HTC)

% Constants and Conversions
g       = 9.81;                 % Gravitational acceleration [m/s^2]
A_ht    = pi*L*D;                  % Heat transfer area
V       = L*pi*D^2/4;              % Volume
C_wall  = M_wall*Cp_wall;          % Heat Capacitance (kJ/K)
C_wall  = 1000*C_wall;             % Covnert heat capacitance from kJ/K to J/K
Q_load  = 1000*Q_load;             % Convert load from kW to W
Cp      = 1000*Cp;                 % Convert Cp from J/g*K to J/kg*K
k       = 1000*k;                  % Convert k from kW/m*K to W/m*K

% Parse states
T       = x(1);                 % Temperature of the tank
P       = x(2);                 % Pressure at bottom of the tank
Tw      = x(3);                 % Wall temperature

% Additional intermediate variable calculations
dP      = (P_in-P)*1000;        % Pressure difference [Pa]
dP      = dP + Rho*g*dH;        % Pressure differential corrected for hieght
um      = sign(dP)*sqrt_Lip(2*abs(dP)/(Rho*(f*L/D+KL)));    % Fluid velocity [m/s]
Re      = Rho*um*D/mu;          % Reynolds number
Pr      = Cp*mu/k;              % Prandtl number (see Incropera, Table 6.2)

if HTC_method == 0
    if Re < 2300
        Nu = 3.66; % (see Incropera, Eq. 8.55)
    else
        Nu = (f/8)*(Re-1000)*Pr / (1+12.7*(f/8)^.5*(Pr^(2/3)-1)); % (see Incropera, Eq. 8.62)  
    end
    H  = PAF*Nu*k/D;            % Heat transfer coefficient (see Incropera, Table 6.2)
else
    H = HTC; 
    % modified by JK 11/11/17
    % H = HTC*Mdot;
end

% Calculate state derivatives
T_dot   = (Mdot*(T_in-T)+H*A_ht/Cp*(Tw-T))/(V*Rho);     % Outlet temperature 
P_dot   = (Mdot-Mdot_down)/(V*Rho*(1/E_fluid+D*(1-v/2)/(t*E))); % Outlet pressure
Tw_dot  = (Q_load - H*A_ht*(Tw-T))/C_wall;              % Wall temperature

% Mux state derivatives
x_dot  = [T_dot,P_dot,Tw_dot];

end

== matlab function DAEMOT_Lib/Thermal/Cold_Plate/Mdot ==
  data: P_in input; P_out input; Mdot output; Rho input; f parameter; D parameter; L parameter; KL parameter; dH parameter
function Mdot = Mdot(P_in,P_out,Rho,f,D,L,KL,dH)

% Constants and Conversions
g           = 9.81;                 % Gravitational acceleration [m/s^2]
A_cross     = pi*D^2/4;             % Cross sectional area
dP          = (P_in-P_out)*1000;    % Pressure differential [Pa]
dP          = dP + Rho*g*dH;        % Pressure differential corrected for hieght
um          = max(0,sign(dP)*sqrt_Lip(2*abs(dP)/(Rho*(f*L/D+KL))));    % Fluid velocity [m/s]

% Calculate outputs
Mdot        = um*Rho*A_cross;       % Mass flow rate [kg/s]

end

== matlab function DAEMOT_Lib/Legacy Components/Flow Split_Junction_Wall/Dynamic_Flow_Split_Junction ==
  data: x input; Mdot_in input; Mdot_out input; T_in input; x_dot output; D parameter; L parameter; t parameter; E parameter; v parameter; rho input; E_fluid input; Q_load input; mu input; k input; Cp input; Rho input; PAF parameter; HTC parameter; HTC_method parameter; Cp_wall parameter; M_wall parameter; A_ht parameter; f parameter
function x_dot  = Dynamic_Flow_Split_Junction(x,Mdot_in,Mdot_out,T_in,D,L,t,E,v,rho,E_fluid,Q_load,mu,k,Cp,Rho,PAF,HTC,HTC_method,Cp_wall,M_wall,A_ht,f)

% Constants and Conversions
Mdot_in_tot   = sum(Mdot_in);     % Total mass flow rate in
Mdot_out_tot  = sum(Mdot_out);    % Total mass flow rate out
V             = pi*D^2/4*L;       % Volume
C_wall        = M_wall*Cp_wall;   % Heat Capacitance (kJ/K)
C_wall        = 1000*C_wall;      % Covnert heat capacitance from kJ/K to J/K
Q_load        = 1000*Q_load;      % Convert load from kW to W
Cp            = 1000*Cp;          % Convert Cp from J/g*K to J/kg*K
k             = 1000*k;           % Convert k from kW/m*K to W/m*K
A_cross       = pi*D^2/4;         % Cross sectional area

% Parse states
T      = x(1);                  % Temperature of the tank
P      = x(2);                  % Pressure at bottom of the tank
Tw     = x(3);                  % Wall temperature

% Additional intermediate variable calculations
um      = Mdot_out_tot/(Rho*A_cross);
Re      = Rho*um*D/mu;          % Reynolds number
Pr      = Cp*mu/k;              % Prandtl number (see Incropera, Table 6.2)

if HTC_method == 0
    if Re < 2300
        Nu = 3.66; % (see Incropera, Eq. 8.55)
    else
        Nu = (f/8)*(Re-1000)*Pr / (1+12.7*(f/8)^.5*(Pr^(2/3)-1)); % (see Incropera, Eq. 8.62)  
    end
    H  = PAF*Nu*k/D;            % Heat transfer coefficient (see Incropera, Table 6.2)
else
    H = HTC; 
    % modified by JK 11/11/17
    % H = HTC*Mdot_out_tot;
end

% Calculate state derivatives
T_dot  = (H*A_ht/Cp*(Tw-T) + (dot(Mdot_in,T_in)-sum(Mdot_out)*T))/(rho*V);  % Split/Junc temperature
P_dot  = (Mdot_in_tot-Mdot_out_tot)/(V*rho*(1/E_fluid+D*(1-v/2)/(t*E))); % Split/Junc pressure
Tw_dot = (Q_load - H*A_ht*(Tw-T))/C_wall;              % Wall temperature

% Mux state derivatives
x_dot  = [T_dot,P_dot,Tw_dot];

end

== matlab function DAEMOT_Lib/Legacy Components/Wall/Wall ==
  data: Q_load input; x_dot output; Q_fluid input; Cp_wall parameter; M_wall parameter
function x_dot   = Wall(Q_load,Q_fluid,Cp_wall,M_wall)

% Constants and Conversions
C_wall  = M_wall*Cp_wall;          % Heat Capacitance (kJ/K)
C_wall  = 1000*C_wall;             % Covnert heat capacitance from kJ/K to J/K
Q_load  = 1000*Q_load;             % Convert load from kW to W
Q_fluid = 1000*Q_fluid;            % Convert load from kW to W

% Calculate state derivatives
Tw_dot  = (Q_load - sum(Q_fluid))/C_wall;  % Wall temperature

% Mux state derivatives
x_dot  = Tw_dot;

end

== matlab function DAEMOT_Lib/Legacy Components/Pipe_P_to_M_Wall/Mdot ==
  data: P_in input; P_out input; Mdot output; Rho input; f parameter; D parameter; L parameter; KL parameter; dH parameter
function Mdot = Mdot(P_in,P_out,Rho,f,D,L,KL,dH)

% Constants and Conversions
g           = 9.81;                 % Gravitational acceleration [m/s^2]
A_cross     = pi*D^2/4;             % Cross sectional area
dP          = (P_in-P_out)*1000;    % Pressure differential [Pa]
dP          = dP + Rho*g*dH;        % Pressure differential corrected for hieght
um          = max(0,sign(dP)*sqrt_Lip(2*abs(dP)/(Rho*(f*L/D+KL))));    % Fluid velocity [m/s]

% Calculate outputs
Mdot        = um*Rho*A_cross;       % Mass flow rate [kg/s]

end

== matlab function DAEMOT_Lib/Legacy Components/Pipe_P_to_M_Wall/Pipe_P_to_M ==
  data: x_dot output; x input; T_in input; Mdot_down input; Mdot input; E_fluid input; D parameter; L parameter; t parameter; E parameter; v parameter; HTC parameter; HTC_method parameter; A_ht parameter; mu input; k input; Cp input; Rho input; T_wall input; Q_kW output; PAF parameter; f parameter
function [x_dot,Q_kW] = Pipe_P_to_M(x,T_in,Mdot_down,Mdot,E_fluid,D,L,t,E,v,HTC,HTC_method,A_ht,mu,k,Cp,Rho,T_wall,PAF, f)

% Constants and Conversions
V       = L*pi*D^2/4;       % Volume
Cp      = 1000*Cp;          % Convert Cp from J/g*K to J/kg*K
k       = 1000*k;           % Convert k from kW/m*K to W/m*K
A_cross = pi*D^2/4;         % Cross sectional area

% Parse states
T       = x(1);                 % Temperature at the outlet of pipe
P       = x(2);                 % Pressure at the outlet of pipe

% Additional intermediate variable calculations
um      = Mdot/(Rho*A_cross);
Re      = Rho*um*D/mu;          % Reynolds number
Pr      = Cp*mu/k;              % Prandtl number (see Incropera, Table 6.2)

if HTC_method == 0
    if Re < 2300
        Nu = 3.66; % (see Incropera, Eq. 8.55)
    else
        Nu = (f/8)*(Re-1000)*Pr / (1+12.7*(f/8)^.5*(Pr^(2/3)-1)); % (see Incropera, Eq. 8.62)  
    end
    H  = PAF*Nu*k/D;            % Heat transfer coefficient (see Incropera, Table 6.2)
else
    H = HTC; 
    % modified by JK 11/11/17
    % H = HTC*Mdot_out_tot;
end

Q = H*A_ht*(T_wall-T);

% Calculate state derivatives
T_dot = ((Q/Cp) + Mdot*(T_in-T))/(V*Rho);  % Pipe outlet temperature
P_dot = (Mdot-Mdot_down)/(V*Rho*(1/E_fluid+D*(1-v/2)/(t*E)));   % Pipe outlet pressure

% Mux state derivatives
x_dot  = [T_dot,P_dot];

Q_kW = Q/1000; % Convert from W to kW

end

== matlab function DAEMOT_Lib/Electrical/Ultracapacitor/Electrical ==
  data: V_t input size=1; V_ci_dot output size=1; V_ci input; V_cd input; V_cl input; props input; V_cd_dot output; V_cl_dot output; I_t output; Q_dot output; Ns parameter; Np parameter
function [V_ci_dot,V_cd_dot,V_cl_dot,I_t,Q_dot] = SC_Electrical(V_t,V_ci,V_cd,V_cl,props,Ns, Np)

%constants
%   only two are kinda wrong
R_i=props(1)/Np;
C_i0=props(2)*Np;
K_c=props(3)*Np;
R_d=props(4)/Np;
C_d=props(5)*Np;
R_l=props(6)/Np;
C_l=props(7)*Np;
R_leak=props(8)/Np;
ESR=.015*Ns/Np;   %ballpark

I_leak=V_t/(Ns*R_leak);
I_i=1/R_i*(V_ci-V_t/Ns);
V_ci_dot=-I_i/(C_i0+K_c*V_ci);
I_l=1/R_l*(V_cl-V_t/Ns);
V_cl_dot=-I_l/C_l;
I_d=1/R_d*(V_cd-V_t/Ns);
V_cd_dot=-I_d/C_d;
I_t=I_i+I_d+I_l-I_leak;

%% Heat Generation
Q_dot=I_leak^2*R_leak+I_i^2*R_i+I_l^2*R_l+I_d^2*R_d+I_t^2*ESR;
%ignoring entropic heat bc smol

== matlab function DAEMOT_Lib/Electrical/Ultracapacitor/Thermal ==
  data: T_c input; T_c_dot output; T_s input; Q_dot input; T_s_dot output; C_c parameter; R_cond parameter; C_s parameter; Q_sink input
function [T_c_dot,T_s_dot] = SC_Thermal(T_c,T_s,Q_dot,C_c,R_cond,C_s,Q_sink)
T_c_dot=1/C_c*(Q_dot+(T_s-T_c)/R_cond);
T_s_dot=1/C_s*(-Q_sink-(T_s-T_c)/R_cond);
